simulink model "WindowFunctionStream_Ex1"  (R2025a)
settings: Solver=VariableStepAuto  StartTime=0.0  StopTime=0.3  RelTol=1e-3
undefined symbols (not defined in the file): None, S, vsva2197, xcvc1902
libraries: aieUtilities x2, dspsrcs4 x1, vmcUtilities x1, aieDSP x1
settings Model: Creator=sdegala  LastModifiedBy=robg
settings ModelReferenceCC: EnableRefExpFcnMdlSchedulingChecks=on
settings RTWCC: GPUComputeCapability=3.5

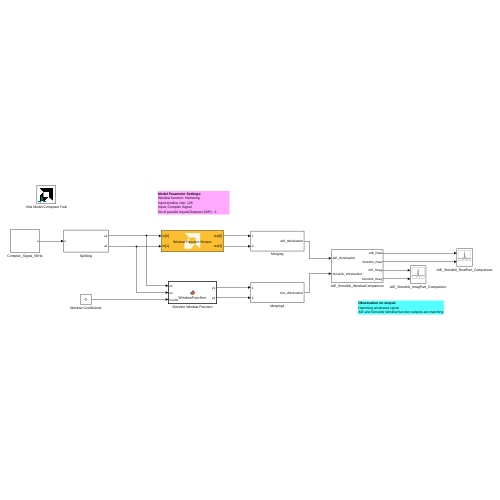
[thumbnail: Simulink's stored preview of the top-level diagram]
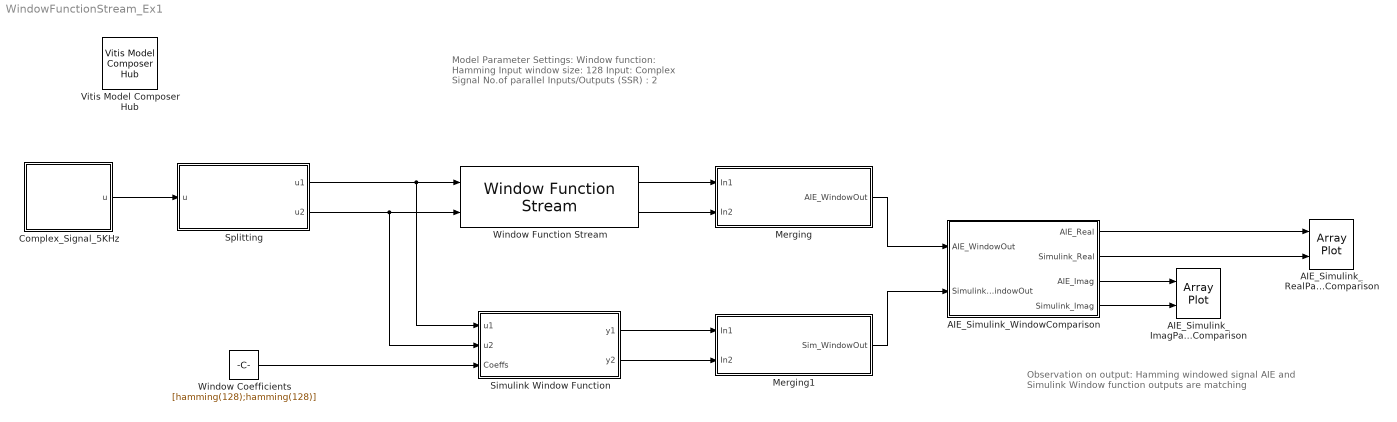
== system WindowFunctionStream_Ex1 ==
  note: Model Parameter Settings:
      | Window function: Hamming
      | Input window size: 128
      | Input: Complex Signal
      | No.of parallel Inputs/Outputs (SSR) : 2
  note: Observation on output:
      | Hamming windowed signal
      | AIE and Simulink Window function outputs are matching
  AIE_Simulink_ImagPart_Comparison : ArrayPlot  NumInputPorts=2  WindowPosition=[5.000000,269.000000,845.000000,423.000000,]  PlotType=Line  AxesScaling=Manual  YLimits=[-4,4]  ShowLegend=on
  AIE_Simulink_RealPart_Comparison : ArrayPlot  NumInputPorts=2  WindowPosition=[5.000000,41.000000,1272.000000,651.000000,]  PlotType=Line  AxesScaling=Manual  YLimits=[-4,4]  ShowLegend=on
  AIE_Simulink_WindowComparison : Subsystem
  Complex_Signal_5KHz : Subsystem
  Merging : Subsystem
  Merging1 : Subsystem
  Simulink Window Function : MATLAB Function  TreatAsAtomicUnit=on
  Splitting : Subsystem
  Vitis Model Composer Hub : vmcUtilities/Vitis Model Composer Hub  Tag=genX  CodeGeneration=off  StartColumn=1  NumberOfColumns=1  TargetDirectory=./code  exportDesign=off  analyzeDesign=off  validateDesignOnHw=off  ExportType=AI Engines  IpVendor=xilinx.com  IpLibrary=hls  IpVersion=1.0  IpHWLanguage=Verilog  AieCompilerOptions={}  AieSimulatorOptions={}  CreateTestbench=off  TestbenchStackSize=10  RunRtlSim=off  RunCSim=off  RunAieSim=off  enableSimulationTimeout=on  enableGraphIterations=on  AieSimTimeout=50000  AieGraphIterations=-1  RunAieSimProfiling=off  LaunchVitisAnalyzer=off  PlotOutput=off  RunX86Sim=off  X86SimTimeout=10  GenHwImage=off  GenLibadfXo=off  GenHwValidationCode=off  PlatformType=Not Specified  HwSystemType=Baremetal  HwValidationTarget=hw  ProjDevice=xcvc1902-vsva2197-1LP-e-S  ProjDevicePart=xcvc1902-vsva2197-1LP-e-S  AIEType=AIE  SamplePeriod=-1  ClockFrequency=200  DataPathParallelism=1  xilinxfamily=versalaicore  part=xcvc1902  speed=-1LP-e-S  package=vsva2197  directory=./netlist  testbench=off  incr_netlist=off  synthesis_tool=Vivado  clock_wrapper=Clock Enables  dbl_ovrd=According to Block Masks  dcm_input_clock_period=10  sysclk_period=10  simulink_period=1  eval_field=0  LogFileName=''  NThreads=4
  Window Coefficients : Constant  Value=[hamming(128);hamming(128)]  OutDataTypeStr=single
  Window Function Stream : aieDSP/Window Function Stream  data_type=cfloat  coeff_type=float  coeff=hamming(128)  point_size=128  is_dyn_pt_size=off  input_window_size=128  shift_val=0  ssr=2  rnd_mode=Floor  sat_mode=0-None  AIE_VARIANT=1  TP_API=1  blockJsonConstraints=[]  blockJsonConstraintsInternal=[]  spec=vmc_stream_fft_window.json  SerializedMaskParamNames=[]  SerializedMaskParamValues=[]  SerializedMaskParamVisibilities=[]  block_type=Window Function Stream  SerializedMaskParamDataypes=typename|typename|coeff_type|uint|uint|uint|uint|uint|uint|uint|uint|uint  SerializedMaskParamEnumStrArr=0|0|0|0|0|0|0|0|Floor,Ceiling,Round to positive infinity,Round to negative infinity,Round symmetrical to infinity,Round symmetrical to zero,Round convergent to even,Round convergent to odd|0-None,1-Asymmetric,3-Symmetric|0|0  SerializedMaskParamEnumValArr=0|0|0|0|0|0|0|0|0,1,2,3,4,5,6,7|0,1,3|0|0  SerializedMaskParamVectorArr=0|0|1|0|0|0|0|0|0|0|0|0  SerializedMaskParamKeys=TT_DATA|TT_COEFF|weights|TP_POINT_SIZE|TP_DYN_PT_SIZE|TP_WINDOW_VSIZE|TP_SHIFT|TP_SSR|TP_RND|TP_SAT|AIE_VARIANT|TP_API
  wires:
  AIE_Simulink_WindowComparison/4(Simulink_Imag) -> AIE_Simulink_ImagPart_Comparison/2
  Complex_Signal_5KHz/1(u) -> Splitting/1(u)
  Window Function Stream/2 -> Merging/2(In2)
  Window Function Stream/1 -> Merging/1(In1)
  Splitting/1(u1) -> Simulink Window Function/1(u1), Window Function Stream/1
  AIE_Simulink_WindowComparison/1(AIE_Real) -> AIE_Simulink_RealPart_Comparison/1
  Simulink Window Function/1(y1) -> Merging1/1(In1)
  Simulink Window Function/2(y2) -> Merging1/2(In2)
  Splitting/2(u2) -> Simulink Window Function/2(u2), Window Function Stream/2
  Merging1/1(Sim_WindowOut) -> AIE_Simulink_WindowComparison/2(Simulink_WindowOut)
  AIE_Simulink_WindowComparison/3(AIE_Imag) -> AIE_Simulink_ImagPart_Comparison/1
  Window Coefficients/1 -> Simulink Window Function/3(Coeffs)
  AIE_Simulink_WindowComparison/2(Simulink_Real) -> AIE_Simulink_RealPart_Comparison/2
  Merging/1(AIE_WindowOut) -> AIE_Simulink_WindowComparison/1(AIE_WindowOut)

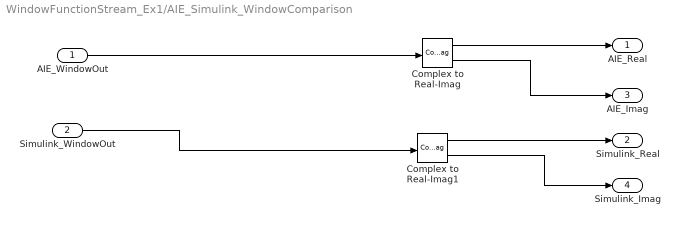
== system WindowFunctionStream_Ex1/AIE_Simulink_WindowComparison ==
  AIE_WindowOut : Inport
  Simulink_WindowOut : Inport  Port=2
  Complex to Real-Imag : ComplexToRealImag
  Complex to Real-Imag1 : ComplexToRealImag
  AIE_Real : Outport
  Simulink_Real : Outport  Port=2
  AIE_Imag : Outport  Port=3
  Simulink_Imag : Outport  Port=4
  wires:
  Complex to Real-Imag1/2 -> Simulink_Imag/1
  Complex to Real-Imag1/1 -> Simulink_Real/1
  AIE_WindowOut/1 -> Complex to Real-Imag/1
  Simulink_WindowOut/1 -> Complex to Real-Imag1/1
  Complex to Real-Imag/1 -> AIE_Real/1
  Complex to Real-Imag/2 -> AIE_Imag/1

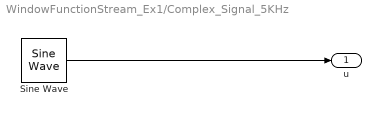
== system WindowFunctionStream_Ex1/Complex_Signal_5KHz ==
  Sine Wave : dspsrcs4/Sine Wave  Amplitude=2  Frequency=5e3  Phase=0  SampleMode=Discrete  OutComplex=Complex  CompMethod=Trigonometric fcn  TableSize=Speed  SampleTime=1/20e3  SamplesPerFrame=256  ResetState=Restart at time zero  OutputFrames=off  dataType=single  wordLen=16  udDataType=sfix(16)  fracBitsMode=Best precision  numFracBits=15  OutDataTypeStr=single  LastOutDataTypeStr=single
  u : Outport
  wires:
  Sine Wave/1 -> u/1

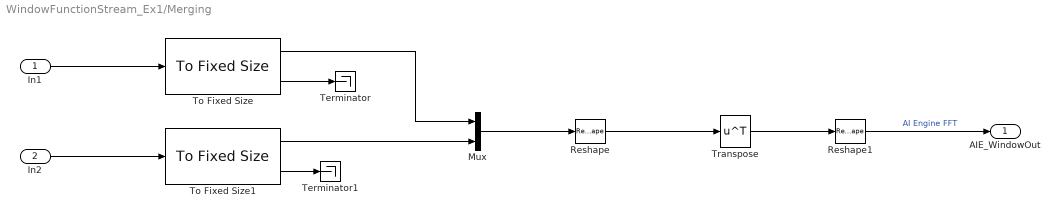
== system WindowFunctionStream_Ex1/Merging ==
  In1 : Inport
  In2 : Inport  Port=2
  Mux : Mux  Inputs=2
  Reshape : Reshape  OutputDimensionality=Customize  OutputDimensions=[128, 2]
  Reshape1 : Reshape  OutputDimensions=[1, 10]
  Terminator : Terminator
  Terminator1 : Terminator
  To Fixed Size : aieUtilities/To Fixed Size  Mode=Produce a valid output signal  OutputSize=Inherit: Same as input  CopyMethod=Buffer samples to form output  HasStatusOutput=on
  To Fixed Size1 : aieUtilities/To Fixed Size  Mode=Produce a valid output signal  OutputSize=Inherit: Same as input  CopyMethod=Buffer samples to form output  HasStatusOutput=on
  Transpose : Math  Operator=transpose
  AIE_WindowOut : Outport
  wires:
  Reshape/1 -> Transpose/1
  To Fixed Size1/2 -> Terminator1/1
  To Fixed Size1/1 -> Mux/2
  In2/1 -> To Fixed Size1/1
  To Fixed Size/2 -> Terminator/1
  Transpose/1 -> Reshape1/1
  To Fixed Size/1 -> Mux/1
  Mux/1 -> Reshape/1
  Reshape1/1 -> AIE_WindowOut/1  "AI Engine FFT"
  In1/1 -> To Fixed Size/1

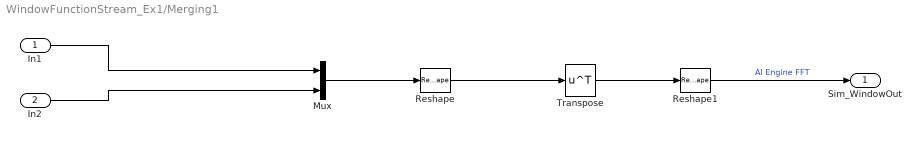
== system WindowFunctionStream_Ex1/Merging1 ==
  In1 : Inport
  In2 : Inport  Port=2
  Mux : Mux  Inputs=2
  Reshape : Reshape  OutputDimensionality=Customize  OutputDimensions=[128, 2]
  Reshape1 : Reshape  OutputDimensions=[1, 10]
  Transpose : Math  Operator=transpose
  Sim_WindowOut : Outport
  wires:
  Reshape/1 -> Transpose/1
  Transpose/1 -> Reshape1/1
  Mux/1 -> Reshape/1
  Reshape1/1 -> Sim_WindowOut/1  "AI Engine FFT"
  In1/1 -> Mux/1
  In2/1 -> Mux/2

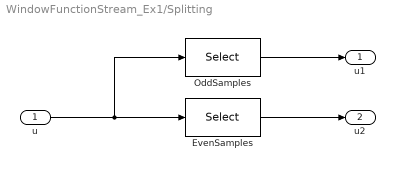
== system WindowFunctionStream_Ex1/Splitting ==
  u : Inport
  EvenSamples : Selector  InputPortWidth=256  IndexOptions=Index vector (dialog)  Indices=2:2:256  OutputSizes=1
  OddSamples : Selector  InputPortWidth=256  IndexOptions=Index vector (dialog)  Indices=1:2:256  OutputSizes=1
  u1 : Outport
  u2 : Outport  Port=2
  wires:
  u/1 -> EvenSamples/1, OddSamples/1
  EvenSamples/1 -> u2/1
  OddSamples/1 -> u1/1

== matlab function WindowFunctionStream_Ex1/Simulink Window Function ==
  data: u1 input; y1 output; u2 input; Coeffs input; y2 output
function [y1,y2] = WindowFunction(u1,u2,Coeffs)
y1 = complex(zeros(128,1,'single'));
y2 = complex(zeros(128,1,'single'));
count = 0;
count2 = 0;
for i = 1:1:256
   if(rem(i,2)==1)
   count = count + 1;
   y1(count,1) = (Coeffs(i,1)*u1(count,1));
   else
   count2 = count2 + 1;
   y2(count2,1) = (Coeffs(i,1)*u2(count2,1));

   end
end

end
